simulink model "MONZA"  (R2025b)
settings: Solver=VariableStepAuto  StartTime=0.0  StopTime=10.0  RelTol=1e-3
values from neighbouring files (symbols this model uses):
  difficulty = 3    [simulacion_monza_tfm.m]
  Ts = 0.033    [simulacion_monza_tfm.m]
libraries: mpclib x1
settings Model: Creator=lucas  LastModifiedBy=kbs-lucas
settings RTWCC: GPUComputeCapability=3.5

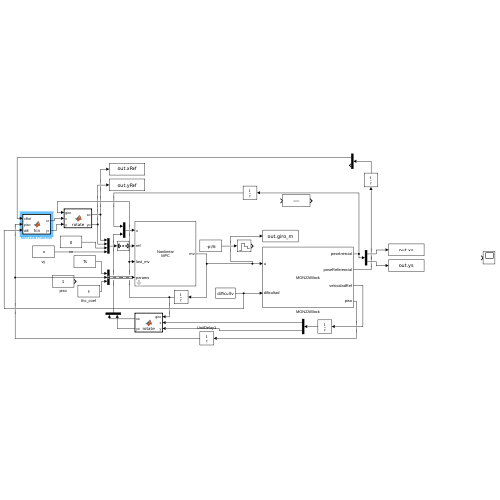
[thumbnail: Simulink's stored preview of the top-level diagram]
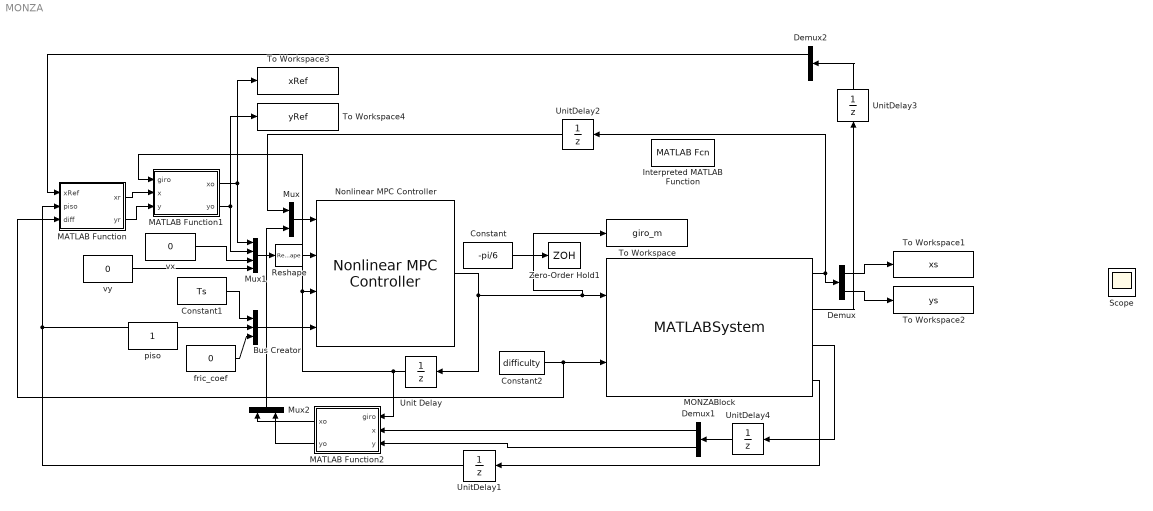
== system MONZA ==
  Bus Creator : BusCreator  Inputs=3  OutDataTypeStr=Bus: myBusObject  NonVirtualBus=on
      settings: InheritFromInputs=off
  Constant : Constant  Value=-pi/6
  Constant1 : Constant  Value=Ts
  Constant2 : Constant  Value=difficulty
  Demux : Demux  Outputs=2
  Demux1 : Demux  Outputs=2
  Demux2 : Demux  Outputs=2
  Interpreted MATLAB Function : MATLABFcn
  MATLAB Function : MATLAB Function  TreatAsAtomicUnit=on
  MATLAB Function1 : MATLAB Function  TreatAsAtomicUnit=on
  MATLAB Function2 : MATLAB Function  TreatAsAtomicUnit=on
  MONZABlock : MATLABSystem  System=MONZABlock  Ts=Ts  disk_mass=0.1  friction_coef=0  SimulateUsing=Code generation
      mask Type: MONZABlock
  Mux : Mux  Inputs=2
  Mux1 : Mux
  Mux2 : Mux  Inputs=2
  Nonlinear MPC Controller : mpclib/Nonlinear MPC Controller  nlmpcobj=controller  UseObjectTs=on  UseMEX=off  md_enabled=off  mvtarget_enabled=off  param_enabled=on  cost_enabled=off  mvseq_enabled=off  stateseq_enabled=off  ovseq_enabled=off  slack_enabled=off  status_enabled=off  ov_min=off  ov_max=off  mv_min=off  mv_max=off  mvrate_min=off  mvrate_max=off  state_min=off  state_max=off  ov_weight=off  mv_weight=off  mvrate_weight=off  ecr_weight=off  nlp_initialize=off
  Reshape : Reshape  OutputDimensionality=Row vector (2-D)
  Scope : Scope
      settings: ActiveDisplayYMinimum=-0.375  ActiveDisplayYMaximum=3.375
  To Workspace : ToWorkspace  VariableName=giro_m  SampleTime=Ts*5
  To Workspace1 : ToWorkspace  VariableName=xs  SampleTime=Ts*5
  To Workspace2 : ToWorkspace  VariableName=ys  SampleTime=Ts*5
  To Workspace3 : ToWorkspace  VariableName=xRef  SampleTime=Ts*5
  To Workspace4 : ToWorkspace  VariableName=yRef  SampleTime=Ts*5
  Unit Delay : UnitDelay  SampleTime=Ts  HasFrameUpgradeWarning=on
  UnitDelay{1..4} (4 alike) : UnitDelay  SampleTime=Ts  HasFrameUpgradeWarning=on
  Zero-Order Hold1 : ZeroOrderHold  SampleTime=Ts*10
  fric_coef : Constant  Value=0
  piso : Constant
  vx : Constant  Value=0
  vy : Constant  Value=0
  wires:
  Demux/1 -> To Workspace1/1
  Demux/2 -> To Workspace2/1
  Constant2/1 -> MONZABlock/2, MATLAB Function/3(diff)
  MONZABlock/1 -> Demux/1, UnitDelay2/1
  MONZABlock/3 -> UnitDelay4/1
  Constant/1 -> Zero-Order Hold1/1
  Reshape/1 -> Nonlinear MPC Controller/2
  fric_coef/1 -> Bus Creator/3
  Mux1/1 -> Reshape/1
  Nonlinear MPC Controller/1 -> To Workspace/1, MONZABlock/1, Unit Delay/1
  Mux/1 -> Nonlinear MPC Controller/1
  Bus Creator/1 -> Nonlinear MPC Controller/4
  vx/1 -> Mux1/3
  MATLAB Function/2(yr) -> MATLAB Function1/3(y)
  MATLAB Function1/2(yo) -> To Workspace4/1, Mux1/2
  Unit Delay/1 -> MATLAB Function1/1(giro), Nonlinear MPC Controller/3, MATLAB Function2/1(giro)
  MATLAB Function/1(xr) -> MATLAB Function1/2(x)
  vy/1 -> Mux1/4
  MATLAB Function1/1(xo) -> To Workspace3/1, Mux1/1
  Constant1/1 -> Bus Creator/1
  MATLAB Function2/2(yo) -> Mux2/2
  MONZABlock/2 -> UnitDelay3/1
  Mux2/1 -> Mux/2
  MATLAB Function2/1(xo) -> Mux2/1
  Demux1/2 -> MATLAB Function2/3(y)
  Demux1/1 -> MATLAB Function2/2(x)
  Demux2/1 -> MATLAB Function/1(xRef)
  MONZABlock/4 -> UnitDelay1/1
  UnitDelay1/1 -> MATLAB Function/2(piso), Bus Creator/2
  UnitDelay2/1 -> Mux/1
  UnitDelay3/1 -> Demux2/1
  UnitDelay4/1 -> Demux1/1

== matlab function MONZA/MATLAB Function1 ==
  data: giro input; x input; xo output; y input; yo output
function [xo,yo] = rotate(giro,x,y)
    xo=x*cos(giro)-y*sin(giro);
    yo=x*sin(giro)+y*cos(giro);
end

== matlab function MONZA/MATLAB Function ==
  data: xRef input; piso input; xr output; diff input; yr output
function [xr, yr] = fcn(xRef,piso,diff)
    piso = int64(piso);
    if mod(piso,int64(2)) == 0
        xRef = xRef - 0.01;
    else
        xRef = xRef + 0.01;
    end
    switch piso
    case 2
        yRot = -0.54 * (xRef * xRef) + 0.0686;
    case 3
        yRot = -0.54 * (xRef * xRef) + 0.03;
    case 4
        yRot = -0.54 * (xRef * xRef) -0.03;
    case 5
        yRot = -0.54 * (xRef * xRef) - 0.0686;
    case 6
        yRot = -0.54 * (xRef * xRef) - 0.1143;
    case 7
        yRot = -0.54 * (xRef * xRef) - 0.16;
    otherwise
        yRot = -0.54 * (xRef * xRef) + 0.1143;
    end
    switch diff
    case 2
        switch piso
            case 2, x = -0.04758; y = 0.06799;
            case 3, x = 0.04969; y = 0.02154;
            case 4, x = -0.04847; y = -0.02411;
            case 5, x = 0.04406; y = -0.06961;
            case 6, x = -0.05409; y = -0.11585;
            case 7, x = -0.02554; y = -0.16035;
            otherwise, x = 0.06211; y = 0.11223;
        end
    case 3
        switch piso
            case 2, x = -0.09503; y = 0.06374;
            case 3, x = 0.09924; y = 0.01759;
            case 4, x = -0.0968; y = -0.02787;
            case 5, x = 0.08803; y = -0.07271;
            case 6, x = -0.108; y = -0.12053;
            case 7, x = -0.02554; y = -0.16035;
            otherwise, x = 0.12394; y= 0.10605;
        end
    otherwise
        switch piso
            case 2, x = 0; y = 0.06857;
            case 3, x = 0; y = 0.02286;
            case 4, x = 0; y = -0.02286;
            case 5, x = 0; y = -0.06857;
            case 6, x = 0; y = -0.11429;
            case 7, x = -0.02554; y = -0.16035;
            otherwise, x = 0; y = 0.11429;
        end
        
    end
    if mod(piso,int64(2)) == 0
        if xRef < x
            xr = x; yr = y;
        else
            xr = xRef; yr = yRot;
        end
    else
        if xRef > x
            xr = x; yr = y;
        else
            xr = xRef; yr = yRot;
        end
    end
    xr = x; yr = y;

== matlab function MONZA/MATLAB Function2 ==
  data: giro input; x input; xo output; y input; yo output
function [xo,yo] = rotate(giro,x,y)
    xo=x*cos(giro)-y*sin(giro);
    yo=x*sin(giro)+y*cos(giro);
end
